simulink model "MPC_control_constraints_Q"  (R2023a)
settings: Solver=VariableStepAuto  StartTime=0.0  StopTime=0.1  RelTol=1e-3
values from neighbouring files (symbols this model uses):
  B_tilda = [sysdis.B(1) Bw_bar(1,1) Bw_bar(1,2); sysdis.B(2) Bw_bar(2,1) Bw_bar(2,2)]    [motor.m]
  D_tilda = [0 0 0 ; 0 0 0]    [motor.m]
  N1 = 100    [motor.m]
  Q1 = [0.001 0; 0 0.001]    [motor.m]
  Q2 = [1 0; 0 1]    [motor.m]
  Q3 = [1000 0; 0 1000]    [motor.m]
  R1 = R_LQ    (= 1)    [motor.m]
  R2 = R_LQ    (= 1)    [motor.m]
  sysdis = c2d(sys,Ts)    [motor.m]
  Ts = 0.001    [parameters.m]
  u_max = 12    [constraints.m]
  u_min = 0    [constraints.m]
  uBar = -(A(1,1)*(-A(2,2)*nref/A(2,1)) + A(1,2)*nref)*L    [motor.m]
  w = [1 1]'    [parameters.m]
  x0 = [0.2 70.3]'    [motor.m]
  yref = [iref nref]'    [motor.m]
undefined symbols (not defined in the file or in its folder): motor_mpc_unconstrained, Sd
settings Model: Creator=margheritamilani  LastModifiedBy=margheritamilani

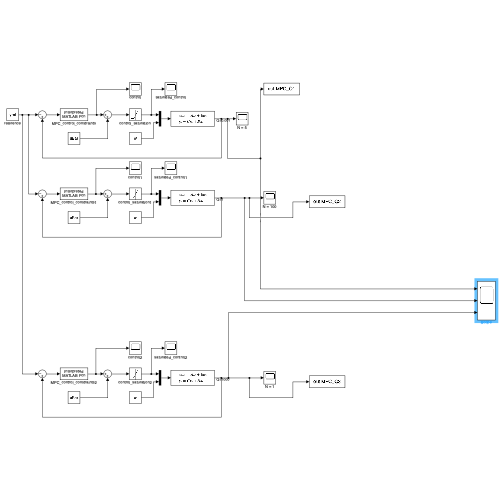
[thumbnail: Simulink's stored preview of the top-level diagram]
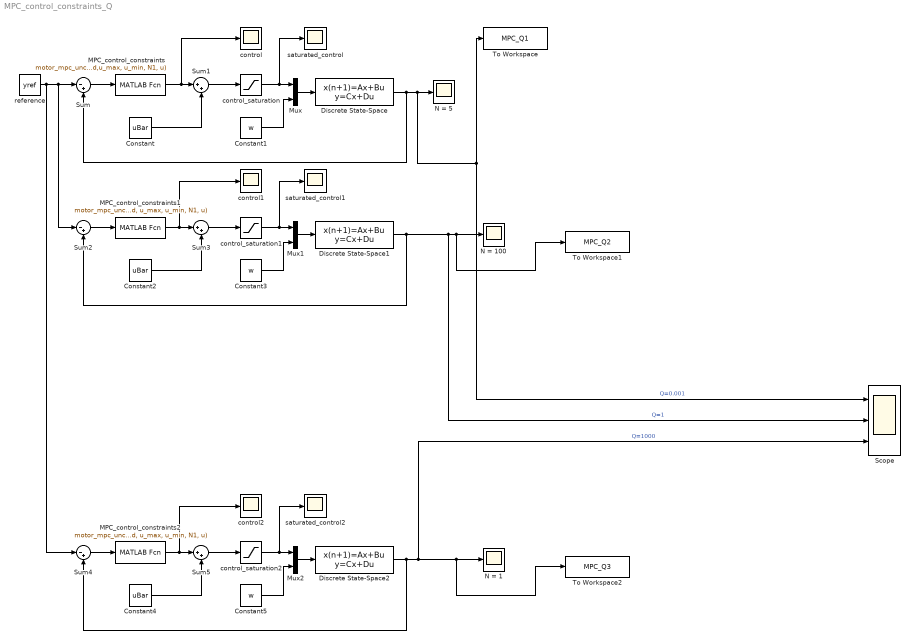
== system MPC_control_constraints_Q ==
  Constant : Constant  Value=uBar
  Constant1 : Constant  Value=w
  Constant2 : Constant  Value=uBar
  Constant3 : Constant  Value=w
  Constant4 : Constant  Value=uBar
  Constant5 : Constant  Value=w
  Discrete State-Space : DiscreteStateSpace  A=sysdis.A  B=B_tilda  C=sysdis.C  D=D_tilda  InitialCondition=x0  SampleTime=Ts
  Discrete State-Space1 : DiscreteStateSpace  A=sysdis.A  B=B_tilda  C=sysdis.C  D=D_tilda  InitialCondition=x0  SampleTime=Ts
  Discrete State-Space2 : DiscreteStateSpace  A=sysdis.A  B=B_tilda  C=sysdis.C  D=D_tilda  InitialCondition=x0  SampleTime=Ts
  MPC_control_constraints : MATLABFcn  MATLABFcn=motor_mpc_unconstrained(sysdis.A, sysdis.B, Q1, R1, Sd,u_max, u_min, N1, u)  OutputDimensions=1
  MPC_control_constraints1 : MATLABFcn  MATLABFcn=motor_mpc_unconstrained(sysdis.A, sysdis.B, Q2, R2, Sd, u_max, u_min, N1, u)  OutputDimensions=1
  MPC_control_constraints2 : MATLABFcn  MATLABFcn=motor_mpc_unconstrained(sysdis.A, sysdis.B, Q3, R2, Sd, u_max, u_min, N1, u)  OutputDimensions=1
  Mux : Mux  Inputs=2
  Mux1 : Mux  Inputs=2
  Mux2 : Mux  Inputs=2
  N = 1 : Scope
  N = 100 : Scope
  N = 5 : Scope
  Scope : Scope  NumInputPorts=3
  Sum : Sum  Inputs=|-+
  Sum1 : Sum  Inputs=|++
  Sum2 : Sum  Inputs=|-+
  Sum3 : Sum  Inputs=|++
  Sum4 : Sum  Inputs=|-+
  Sum5 : Sum  Inputs=|++
  To Workspace : ToWorkspace  VariableName=MPC_Q1  SaveFormat=Timeseries  SampleTime=-1
  To Workspace1 : ToWorkspace  VariableName=MPC_Q2  SaveFormat=Timeseries  SampleTime=-1
  To Workspace2 : ToWorkspace  VariableName=MPC_Q3  SaveFormat=Timeseries  SampleTime=-1
  control : Scope
  control1 : Scope
  control2 : Scope
  control_saturation : Saturate  UpperLimit=u_max  LowerLimit=u_min
  control_saturation1 : Saturate  UpperLimit=u_max  LowerLimit=u_min
  control_saturation2 : Saturate  UpperLimit=u_max  LowerLimit=u_min
  reference : Constant  Value=yref
  saturated_control : Scope
  saturated_control1 : Scope
  saturated_control2 : Scope
  wires:
  Sum/1 -> MPC_control_constraints/1
  Constant2/1 -> Sum3/2
  Sum1/1 -> control_saturation/1
  Discrete State-Space/1 -> To Workspace/1, Scope/1, N = 5/1, Sum/2  "Q=0.001"
  MPC_control_constraints/1 -> control/1, Sum1/1
  control_saturation1/1 -> saturated_control1/1, Mux1/1
  Sum3/1 -> control_saturation1/1
  control_saturation/1 -> saturated_control/1, Mux/1
  MPC_control_constraints1/1 -> control1/1, Sum3/1
  Mux/1 -> Discrete State-Space/1
  Constant/1 -> Sum1/2
  Constant3/1 -> Mux1/2
  Mux1/1 -> Discrete State-Space1/1
  Sum2/1 -> MPC_control_constraints1/1
  Constant1/1 -> Mux/2
  Discrete State-Space1/1 -> Scope/2, To Workspace1/1, N = 100/1, Sum2/2  "Q=1"
  Constant4/1 -> Sum5/2
  reference/1 -> Sum4/1, Sum2/1, Sum/1
  Discrete State-Space2/1 -> Scope/3, To Workspace2/1, N = 1/1, Sum4/2  "Q=1000"
  Sum4/1 -> MPC_control_constraints2/1
  MPC_control_constraints2/1 -> control2/1, Sum5/1
  control_saturation2/1 -> saturated_control2/1, Mux2/1
  Sum5/1 -> control_saturation2/1
  Mux2/1 -> Discrete State-Space2/1
  Constant5/1 -> Mux2/2
